simulink subsystem "InversePendulum"  (R2022b)
settings: Solver=VariableStepAuto  StartTime=0.0  StopTime=10.0  RelTol=1e-3
undefined symbols (not defined in the file): A, B, g, I, Init_St, l, m, M, p
settings Model: Creator=Лиза  LastModifiedBy=Лиза
settings OptimizationCC: ReuseModelBlockBuffer=on

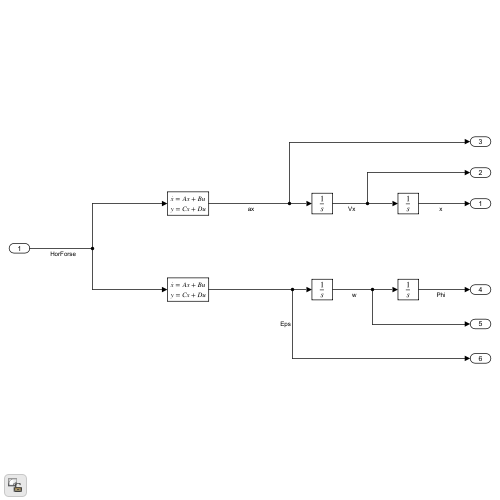
[thumbnail: Simulink's stored preview of the top-level diagram]
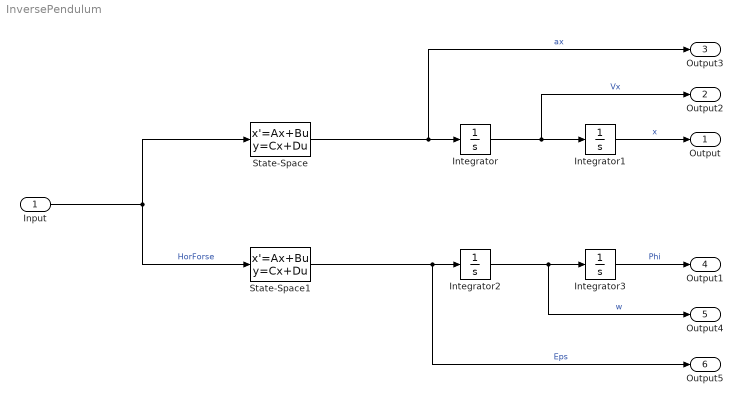
== system InversePendulum ==
  Input : Inport
  Integrator{,1..3} (4 alike) : Integrator
  State-Space : StateSpace  A=A  B=B  C="[ 0      0          (m^2*g*l^2)/p   0]"  D=[(I+m*l^2)/p]  InitialCondition=Init_St
  State-Space1 : StateSpace  A=A  B=B  C=[ 0 0 m*g*l*(M+m)/p 0]  D=m*l/p  InitialCondition=Init_St
  Output : Outport
  Output2 : Outport  Port=2
  Output3 : Outport  Port=3
  Output1 : Outport  Port=4
  Output4 : Outport  Port=5
  Output5 : Outport  Port=6
  wires:
  Input/1 -> State-Space1/1, State-Space/1  "HorForse"
  State-Space/1 -> Output3/1, Integrator/1  "ax"
  Integrator/1 -> Output2/1, Integrator1/1  "Vx"
  State-Space1/1 -> Output5/1, Integrator2/1  "Eps"
  Integrator2/1 -> Output4/1, Integrator3/1  "w"
  Integrator1/1 -> Output/1  "x"
  Integrator3/1 -> Output1/1  "Phi"
